simulink model "CPS_PowerSync_System"  (R2024a)
settings: Solver=FixedStepAuto  StartTime=0.0  StopTime=50  FixedStep=0.1  RelTol=1e-3
model workspace (MAT data in the model file):
  SoC : Simulink.Signal (value not decoded)
undefined symbols (not defined in the file or in its folder): m, v_CP1, v_CP2, v_CP3, w_CP1, w_CP2, w_CP3
(part 3 of 3)

== stateflow chart CPS_PowerSync_System/ElecritcVehicles3 ==
  settings: updateMethod=CONTINUOUS  sampleTime=1
  state Normal
    entry:
    % Imposto generatore casuali in dtato basato su ora corrente
    rng("shuffle")
    % Imposto casualmente valore iniziale di SoC
    SoC_EV3 = randi([0,10])/10
    state Unplugged
      state Assigment
    state Plugged
      state Charging
      state Completed
      (default) -> (junction 33)
      (junction 33) -> Charging [order 2]
      (junction 33) -> Completed [order 1] : [SoC_EV3 == 1]
      Completed -> Charging : [SoC_EV3 <= 0.95]
      Charging -> Completed : [SoC_EV3 == 1]
    (default) -> Unplugged
    Unplugged -> Plugged : [runPythonScriptRandGen <= (1 - exp((-(elapsed(sec))/10)))]
    Plugged -> Unplugged : % Il veicolo si scollega e se ne collega un altro
        | % P1: Maggiore è il valore di SoC più è probabile che il veicolo se ne vada
        | % P2: La proabilità che il veicolo se ne vada aumenta con il passare del tempo
        | [runPythonScriptRandGen <= SoC_EV3 && runPythonScriptRandGen <= (1 - exp((-(elapsed(sec))/100)))]
        | {% Arriva nuovo veicolo con un proprio valore di SoC
        |  SoC_EV3 = randi([0,10])/10}
  (default) -> Normal
  data: sf_internal_action_state_placeholder_data local double size=1 =0; randUniform function_output; sf_internal_action_state_placeholder_data local double size=1 =0; sf_internal_action_state_placeholder_data local double size=1 =0; powerFlow input double; powerRequest output boolean =0; plug output boolean size=1; SoC_EV3 data_store_memory
  function randUniform = runPythonScriptRandGen:
    | function randUniform = runPythonScriptRandGen()
    | 
    |     % La funzione è estrinseca, cioè non verrà compilata in codice C.
    |     % Deve essere eseguita come una chiamata MATLAB normale.
    |     coder.extrinsic('pyrunfile');
    | 
    |     % Inizializzo la variabile
    |     randUniform = 0;
    | 
    |     % Esegue lo script Python rand.py e cattura il risultato.
    |     randUniform = pyrunfile("rand.py", "r");
    | 
    | end

== matlab function CPS_PowerSync_System/ElecritcVehicles3/Normal.Plugged.Charging/If Action Subsystem/MATLAB Function ==
  data: y output; SoC_EV3 data_store_memory
function y = fcn

global SoC_EV3

y = SoC_EV3;

== matlab function CPS_PowerSync_System/ElecritcVehicles3/Normal.Plugged.Charging/If Action Subsystem/MATLAB Function1 ==
  settings: updateMethod=DISCRETE
  data: SoC_EV3 data_store_memory; u_current input
function fcn(u_current)

global SoC_EV3

SoC_EV3 = u_current;

== matlab function CPS_PowerSync_System/ElecritcVehicles3/Normal.Plugged.Completed/If Action Subsystem/MATLAB Function ==
  data: y output; SoC_EV3 data_store_memory
function y = fcn

global SoC_EV3

y = SoC_EV3;

== matlab function CPS_PowerSync_System/ElecritcVehicles3/Normal.Plugged.Completed/If Action Subsystem/MATLAB Function1 ==
  settings: updateMethod=DISCRETE
  data: SoC_EV3 data_store_memory; u input
function fcn(u)

global SoC_EV3

SoC_EV3 = u;

== matlab function CPS_PowerSync_System/ElecritcVehicles1/Normal.Plugged.Charging/If Action Subsystem/MATLAB Function1 ==
  settings: updateMethod=DISCRETE
  data: SoC_EV1 data_store_memory; u_current input
function fcn(u_current)

global SoC_EV1

SoC_EV1 = u_current;

== matlab function CPS_PowerSync_System/ElecritcVehicles1/Normal.Plugged.Completed/If Action Subsystem/MATLAB Function ==
  data: y output; SoC_EV1 data_store_memory
function y = fcn

global SoC_EV1

y = SoC_EV1;

== matlab function CPS_PowerSync_System/ElecritcVehicles1/Normal.Plugged.Completed/If Action Subsystem/MATLAB Function1 ==
  settings: updateMethod=DISCRETE
  data: SoC_EV1 data_store_memory; u input
function fcn(u)

global SoC_EV1

SoC_EV1 = u;

== matlab function CPS_PowerSync_System/MATLAB Function ==
  data: y output; SoC_EV1 data_store_memory
function y = fcn

global SoC_EV1

y = SoC_EV1;

== matlab function CPS_PowerSync_System/MATLAB Function1 ==
  data: y output; SoC_EV2 data_store_memory
function y = fcn

global SoC_EV2

y = SoC_EV2;

== matlab function CPS_PowerSync_System/MATLAB Function2 ==
  data: y output; SoC_EV3 data_store_memory
function y = fcn

global SoC_EV3

y = SoC_EV3;
